simulink model "Bias_TestGen15"  (R2017b)
settings: Solver=FixedStepDiscrete  StartTime=0.0  StopTime=10.0  RelTol=1e-3
settings Model: Creator=hbourbou  LastModifiedBy=hbourbou
settings DebuggingCC: ParameterOverflowMsg=none

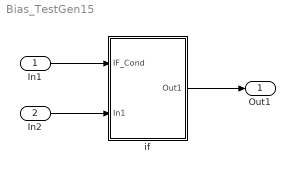
== system Bias_TestGen15 ==
  In1 : Inport
  In2 : Inport  Port=2
  if : Subsystem  AncestorBlock=Block_TestLib/if
  Out1 : Outport
  wires:
  In1/1 -> if/1(IF_Cond)
  In2/1 -> if/2(In1)
  if/1(Out1) -> Out1/1

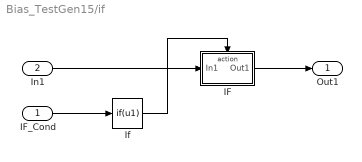
== system Bias_TestGen15/if ==
  IF_Cond : Inport  OutDataTypeStr=boolean
  In1 : Inport  Port=2
  IF : Subsystem  TreatAsAtomicUnit=on
  If : If  IfExpression=u1  ShowElse=off
  Out1 : Outport
  wires:
  If/1 -> IF/Action
  In1/1 -> IF/1(In1)
  IF_Cond/1 -> If/1
  IF/1(Out1) -> Out1/1

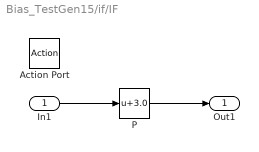
== system Bias_TestGen15/if/IF ==
  In1 : Inport  PortDimensions=1
  Action Port : ActionPort  ActionType=then
  P : Bias  Bias=3.0
  Out1 : Outport
  wires:
  In1/1 -> P/1
  P/1 -> Out1/1
